simulink model "deadReckoning_rover_closedloop_aek"  (R2023a)
settings: Solver=FixedStepAuto  StartTime=0.0  StopTime=25  FixedStep=0.1  RelTol=1e-3  EnableMultiTasking=on
PreLoadFcn:
  | robotParameters;
model workspace (MAT data in the model file):
  axleLength = 0.085
  ticksPerRot = 1200
  wheelR = 0.045
undefined symbols (not defined in the file): DiscIntNeverNeededParam, PWMcmdMonoL, PWMcmdMonoR, speedMonoL, speedMonoR
libraries: arduinomotorcarrierlib x4, M5Core_Library x4, simulink_extras x2, simulink x1, mobileRoboticsTrainingLib x1
settings Model: ExtModeTrigDuration=2  Creator=sseshadr  LastModifiedBy=auw_a
settings SolverCC: AlgebraicLoopSolver=TrustRegion
settings DataIOCC: ReturnWorkspaceOutputs=off
settings OptimizationCC: MaxStackSize=64  EfficientTunableParamExpr=on
settings DebuggingCC: ParameterPrecisionLossMsg=none  ParameterTunabilityLossMsg=error  UnconnectedInputMsg=warning  UnconnectedOutputMsg=warning  UnconnectedLineMsg=warning  ArithmeticOperatorsInVariantConditions=warning
settings HardwareCC: ProdBitPerPointer=32  ProdBitPerSizeT=32  ProdBitPerPtrDiffT=32  ProdLargestAtomicInteger=Long  ProdLargestAtomicFloat=Double  ProdWordSize=32  ProdHWDeviceType=ARM Compatible->ARM Cortex
settings ModelReferenceCC: EnableRefExpFcnMdlSchedulingChecks=on
settings SFSimCC: SimUseLocalCustomCode=off  MATLABDynamicMemAlloc=off  CustomCodeUndefinedFunction=UseInterfaceOnly
settings RTWCC: Description=Embedded Coder  SystemTargetFile=ert.tlc  HardwareBoard=Arduino Nano 33 IoT  TLCOptions="-aInlineSetEventsForThisBaseRateFcn=TLC_FALSE -aSuppressMultiTaskScheduler=TLC_FALSE   -aRateBasedStepFcn=1"  TemplateMakefile=ert_default_tmf  GenerateReport=on  RTWUseLocalCustomCode=off  Toolchain=Arduino ARM  BuildConfiguration=Faster Runs  IncludeHyperlinkInReport=on  LaunchReport=on  GenerateTraceInfo=on  GenerateTraceReport=on  GenerateTraceReportSl=on  GenerateTraceReportSf=on  GenerateTraceReportEml=on  DLArmComputeVersion=19.05
settings CodeAppCC: ForceParamTrailComments=on  IgnoreCustomStorageClasses=off  OperatorAnnotations=on  SimulinkDataObjDesc=on  SFDataObjDesc=on  MATLABFcnDesc=on  InsertBlockDesc=on  StateflowObjectComments=on  MATLABSourceComments=on
settings ERTTargetCC: MultiwordLength=2048  SupportContinuousTime=on  SupportVariableSizeSignals=on  ExtModeTransport=3  ExtModeStaticAlloc=on  ExtModeStaticAllocSize=8192  ExtModeMexFile=ext_xcp  ExtModeIntrfLevel=Level2 - Open

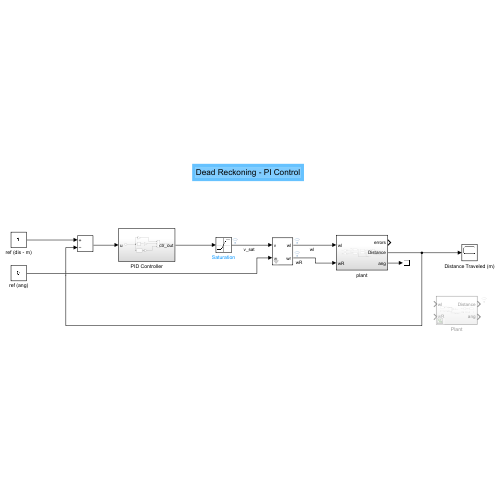
[thumbnail: Simulink's stored preview of the top-level diagram]
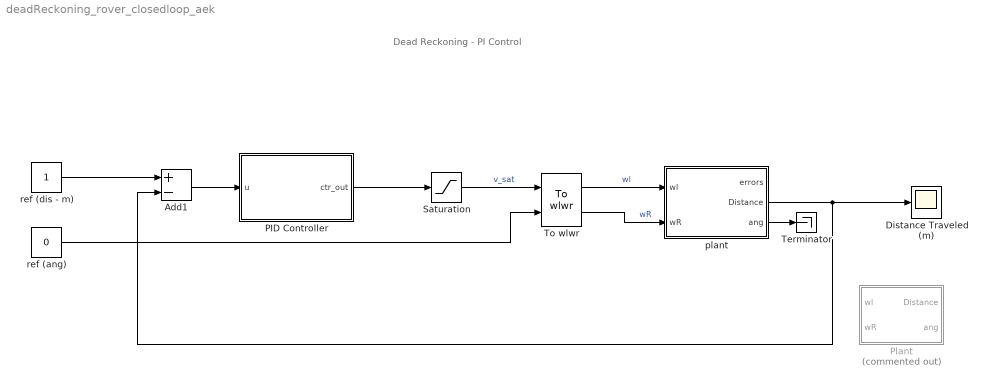
== system deadReckoning_rover_closedloop_aek ==
  note: Dead Reckoning - PI Control
  Add1 : Sum  Inputs=+-
  Distance Traveled (m) : Scope
  PID Controller : Subsystem
  Plant : Subsystem  Commented=on
  Saturation : Saturate  UpperLimit=5  LowerLimit=-5
  Terminator : Terminator
  To wlwr : mobileRoboticsTrainingLib/To wlwr  axleLength=axleLength  wheelR=wheelR
  plant : Subsystem
  ref (ang) : Constant  Value=0
  ref (dis - m) : Constant
  wires:
  Saturation/1 -> To wlwr/1  "v_sat"
  plant/2(Distance) -> Add1/2, Distance Traveled (m)/1
  To wlwr/1 -> plant/1(wl)  "wl"
  ref (dis - m)/1 -> Add1/1
  Add1/1 -> PID Controller/1(u)
  To wlwr/2 -> plant/2(wR)  "wR"
  ref (ang)/1 -> To wlwr/2
  plant/3(ang) -> Terminator/1
  PID Controller/1(ctr_out) -> Saturation/1

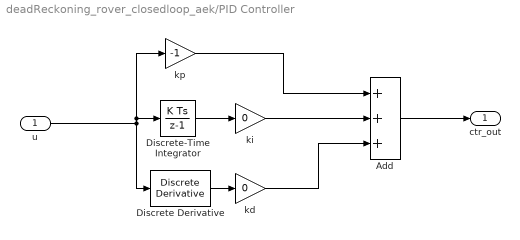
== system deadReckoning_rover_closedloop_aek/PID Controller ==
  u : Inport
  Add : Sum  Inputs=+++
  Discrete Derivative : simulink/Discrete/Discrete Derivative  gainval=1.0  ICPrevScaledInput=0.0  OutMin=[]  OutMax=[]  OutDataType=fixdt(1, 16)  OutScaling=2^-10  DoSatur=off
  Discrete-Time Integrator : DiscreteIntegrator  SampleTime=-1  ICPrevOutput=DiscIntNeverNeededParam  ICPrevScaledInput=DiscIntNeverNeededParam
  kd : Gain  Gain=0
  ki : Gain  Gain=0
  kp : Gain  Gain=-1
  ctr_out : Outport
  wires:
  kp/1 -> Add/1
  kd/1 -> Add/3
  Discrete-Time Integrator/1 -> ki/1
  u/1 -> Discrete-Time Integrator/1, kp/1, Discrete Derivative/1
  Discrete Derivative/1 -> kd/1
  ki/1 -> Add/2
  Add/1 -> ctr_out/1

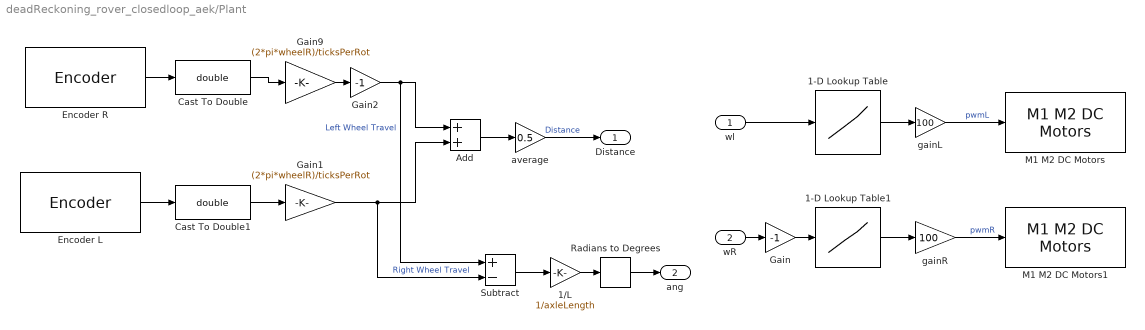
== system deadReckoning_rover_closedloop_aek/Plant ==
  wl : Inport
  wR : Inport  Port=2
  1-D Lookup Table : Lookup_n-D  NumberOfTableDimensions=1  BreakpointsForDimension1=speedMonoL  Table=PWMcmdMonoL  ExtrapMethod=Clip  InternalRulePriority=Speed  RndMeth=Simplest
  1-D Lookup Table1 : Lookup_n-D  NumberOfTableDimensions=1  BreakpointsForDimension1=speedMonoR  Table=PWMcmdMonoR  ExtrapMethod=Clip  InternalRulePriority=Speed  RndMeth=Simplest
  1/L : Gain  Gain=1/axleLength
  Add : Sum  OutDataTypeStr=uint32
  Cast To Double : DataTypeConversion  OutDataTypeStr=double  SaturateOnIntegerOverflow=off  RndMeth=Floor
  Cast To Double1 : DataTypeConversion  OutDataTypeStr=double  SaturateOnIntegerOverflow=off  RndMeth=Floor
  Encoder L : arduinomotorcarrierlib/Encoder  SlaveAddress=uint8( hex2dec( '66' ) )  blockPlatform=ARDUINO  Encoder=2  ShowSpeed=off  ResetOption=on  SampleTime=0.1
  Encoder R : arduinomotorcarrierlib/Encoder  SlaveAddress=uint8( hex2dec( '66' ) )  blockPlatform=ARDUINO  Encoder=1  ShowSpeed=off  ResetOption=on  SampleTime=0.1
  Gain : Gain  Gain=-1
  Gain1 : Gain  Gain=(2*pi*wheelR)/ticksPerRot
  Gain2 : Gain  Gain=-1
  Gain9 : Gain  Gain=(2*pi*wheelR)/ticksPerRot
  M1 M2 DC Motors : arduinomotorcarrierlib/M1 M2 DC Motors  SlaveAddress=uint8( hex2dec( '66' ) )  blockPlatform=ARDUINO  MotorNumber=M2  MotorCarrierPWMFreq=100
  M1 M2 DC Motors1 : arduinomotorcarrierlib/M1 M2 DC Motors  SlaveAddress=uint8( hex2dec( '66' ) )  blockPlatform=ARDUINO  MotorNumber=M1  MotorCarrierPWMFreq=100
  Radians to Degrees : simulink_extras/Transformations/Radians to Degrees
  Subtract : Sum  Inputs=+-  OutDataTypeStr=uint32
  average : Gain  Gain=0.5
  gainL : Gain  Gain=100
  gainR : Gain  Gain=100
  Distance : Outport
  ang : Outport  Port=2
  wires:
  Gain1/1 -> Subtract/2, Add/2  "Right Wheel Travel"
  Encoder L/1 -> Cast To Double1/1
  1-D Lookup Table/1 -> gainL/1
  Gain9/1 -> Gain2/1
  1-D Lookup Table1/1 -> gainR/1
  gainL/1 -> M1 M2 DC Motors/1  "pwmL"
  gainR/1 -> M1 M2 DC Motors1/1  "pwmR"
  Add/1 -> average/1
  Gain/1 -> 1-D Lookup Table1/1
  wl/1 -> 1-D Lookup Table/1
  wR/1 -> Gain/1
  average/1 -> Distance/1  "Distance"
  Subtract/1 -> 1/L/1
  1/L/1 -> Radians to Degrees/1
  Radians to Degrees/1 -> ang/1
  Encoder R/1 -> Cast To Double/1
  Gain2/1 -> Add/1, Subtract/1  "Left Wheel Travel"
  Cast To Double/1 -> Gain9/1
  Cast To Double1/1 -> Gain1/1

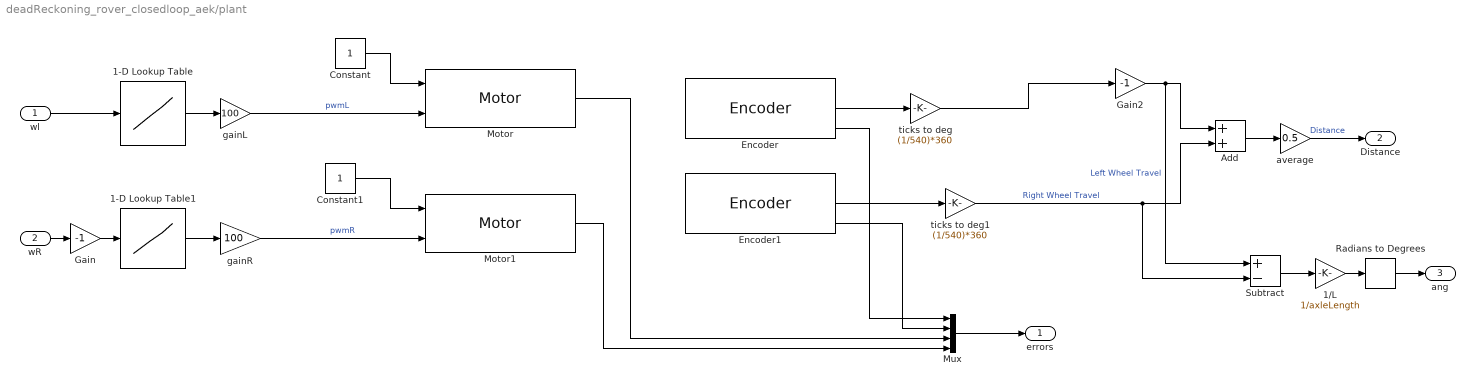
== system deadReckoning_rover_closedloop_aek/plant ==
  wl : Inport
  wR : Inport  Port=2
  1-D Lookup Table : Lookup_n-D  NumberOfTableDimensions=1  BreakpointsForDimension1=speedMonoL  Table=PWMcmdMonoL  ExtrapMethod=Clip  InternalRulePriority=Speed  RndMeth=Simplest
  1-D Lookup Table1 : Lookup_n-D  NumberOfTableDimensions=1  BreakpointsForDimension1=speedMonoR  Table=PWMcmdMonoR  ExtrapMethod=Clip  InternalRulePriority=Speed  RndMeth=Simplest
  1/L : Gain  Gain=1/axleLength
  Add : Sum  OutDataTypeStr=uint32
  Constant : Constant
  Constant1 : Constant
  Encoder : M5Core_Library/Encoder  M5_motor=3  s=0.01
  Encoder1 : M5Core_Library/Encoder  M5_motor=3  s=0.01
  Gain : Gain  Gain=-1
  Gain2 : Gain  Gain=-1
  Motor : M5Core_Library/Motor  M5_motor=M3
  Motor1 : M5Core_Library/Motor  M5_motor=M1
  Mux : Mux
  Radians to Degrees : simulink_extras/Transformations/Radians to Degrees
  Subtract : Sum  Inputs=+-  OutDataTypeStr=uint32
  average : Gain  Gain=0.5
  gainL : Gain  Gain=100
  gainR : Gain  Gain=100
  ticks to deg : Gain  Gain=(1/540)*360
  ticks to deg1 : Gain  Gain=(1/540)*360
  errors : Outport
  Distance : Outport  Port=2
  ang : Outport  Port=3
  wires:
  Mux/1 -> errors/1
  Encoder/2 -> ticks to deg/1
  ticks to deg/1 -> Gain2/1
  Constant/1 -> Motor/1
  Constant1/1 -> Motor1/1
  wl/1 -> 1-D Lookup Table/1
  gainR/1 -> Motor1/2  "pwmR"
  Gain/1 -> 1-D Lookup Table1/1
  gainL/1 -> Motor/2  "pwmL"
  wR/1 -> Gain/1
  1-D Lookup Table1/1 -> gainR/1
  1-D Lookup Table/1 -> gainL/1
  1/L/1 -> Radians to Degrees/1
  average/1 -> Distance/1  "Distance"
  Radians to Degrees/1 -> ang/1
  Add/1 -> average/1
  Gain2/1 -> Add/1, Subtract/1  "Left Wheel Travel"
  Subtract/1 -> 1/L/1
  ticks to deg1/1 -> Subtract/2, Add/2  "Right Wheel Travel"
  Encoder1/2 -> ticks to deg1/1
  Encoder/3 -> Mux/1
  Encoder1/3 -> Mux/2
  Motor/1 -> Mux/3
  Motor1/1 -> Mux/4
